simulink library "tp333079"  (Simulink 5.0)
values from neighbouring files (symbols this model uses):
  b = 1    [main_flock3.m]    (also in main_flock4.m; params_flocking_ros.m)
undefined symbols (not defined in the file or in its folder): AC, AlphaBnd, BetaBnd, CDda, CDde, CDdf, CDdr, CDM, CDmin, CGempty, CGgross, CL0, CLa, CLalphadot, Clbeta, Clda, CLde, CLdf, Cldr, CLM, CLmind, Clp, CLq, Clr, Cm0, Cma, Cmalphadot, Cmde, Cmdf, CmM, Cmq, Cnbeta, Cnda, Cndr, Cnp, Cnr, CP, CT, CYbeta, CYda, CYdr, CYp, CYr, Displacement, dmy, Engine, EulerIni, FuelFlow, FuelIni, J, Jempty, Jeng, Jgross, Jprop, MAC, MAP, MAPLim, MassIni, MaxPower, mempty ... (+26)
libraries: aerosimlib x325, simulink3 x42
(part 8 of 11)

== system tp333079/Unit Conversion/Pressure/inHg2Pa ==
  inHg : Inport  Port=1  PortDimensions=-1  SampleTime=-1  DataType=auto
      settings: SignalType=auto
  Gain : Gain  Gain=1/0.00029529  Multiplication=Element-wise(K.*u)  SaturateOnIntegerOverflow=on
  Pa : Outport  Port=1
  wires:
  inHg/1 -> Gain/1
  Gain/1 -> Pa/1

== system tp333079/Unit Conversion/Temperature/F2K ==
  F : Inport  Port=1  PortDimensions=-1  SampleTime=-1  DataType=auto
      settings: SignalType=auto
  Constant : Constant  Value=459.67
  Gain : Gain  Gain=1/1.8  Multiplication=Element-wise(K.*u)  SaturateOnIntegerOverflow=on
  Sum : Sum  Inputs=|++  SaturateOnIntegerOverflow=on
  K : Outport  Port=1
  wires:
  Constant/1 -> Sum/2
  F/1 -> Sum/1
  Sum/1 -> Gain/1
  Gain/1 -> K/1

== system tp333079/Unit Conversion/Temperature/K2F ==
  K : Inport  Port=1  PortDimensions=-1  SampleTime=-1  DataType=auto
      settings: SignalType=auto
  Constant : Constant  Value=459.67
  Gain : Gain  Gain=1.8  Multiplication=Element-wise(K.*u)  SaturateOnIntegerOverflow=on
  Sum : Sum  Inputs=|+-  SaturateOnIntegerOverflow=on
  F : Outport  Port=1
  wires:
  K/1 -> Gain/1
  Gain/1 -> Sum/1
  Constant/1 -> Sum/2
  Sum/1 -> F/1

== system tp333079/Unit Conversion/Velocity/km/h 2 m/s ==
  In : Inport  Port=1  PortDimensions=-1  SampleTime=-1  DataType=auto
      settings: SignalType=auto
  Gain : Gain  Gain=1/3.6  Multiplication=Element-wise(K.*u)  SaturateOnIntegerOverflow=on
  Out : Outport  Port=1
  wires:
  Gain/1 -> Out/1
  In/1 -> Gain/1

== system tp333079/Unit Conversion/Velocity/kts 2 m/s ==
  In : Inport  Port=1  PortDimensions=-1  SampleTime=-1  DataType=auto
      settings: SignalType=auto
  Gain : Gain  Gain=0.5147902667  Multiplication=Element-wise(K.*u)  SaturateOnIntegerOverflow=on
  Out : Outport  Port=1
  wires:
  Gain/1 -> Out/1
  In/1 -> Gain/1

== system tp333079/Unit Conversion/Velocity/m/s 2 km/h ==
  In : Inport  Port=1  PortDimensions=-1  SampleTime=-1  DataType=auto
      settings: SignalType=auto
  Gain : Gain  Gain=3.6  Multiplication=Element-wise(K.*u)  SaturateOnIntegerOverflow=on
  Out : Outport  Port=1
  wires:
  In/1 -> Gain/1
  Gain/1 -> Out/1

== system tp333079/Unit Conversion/Velocity/m/s 2 kts ==
  In : Inport  Port=1  PortDimensions=-1  SampleTime=-1  DataType=auto
      settings: SignalType=auto
  Gain : Gain  Gain=1.9425386701  Multiplication=Element-wise(K.*u)  SaturateOnIntegerOverflow=on
  Out : Outport  Port=1
  wires:
  In/1 -> Gain/1
  Gain/1 -> Out/1

== system tp333079/Unit Conversion/Velocity/m/s 2 mph ==
  In : Inport  Port=1  PortDimensions=-1  SampleTime=-1  DataType=auto
      settings: SignalType=auto
  Gain : Gain  Gain=2.2369362921  Multiplication=Element-wise(K.*u)  SaturateOnIntegerOverflow=on
  Out : Outport  Port=1
  wires:
  Gain/1 -> Out/1
  In/1 -> Gain/1

== system tp333079/Unit Conversion/Velocity/mph 2 m/s ==
  In : Inport  Port=1  PortDimensions=-1  SampleTime=-1  DataType=auto
      settings: SignalType=auto
  Gain : Gain  Gain=0.44704  Multiplication=Element-wise(K.*u)  SaturateOnIntegerOverflow=on
  Out : Outport  Port=1
  wires:
  In/1 -> Gain/1
  Gain/1 -> Out/1

== system tp333079/Unit Conversion/Volume/gal 2 l ==
  In : Inport  Port=1  PortDimensions=-1  SampleTime=-1  DataType=auto
      settings: SignalType=auto
  Gain : Gain  Gain=3.785412  Multiplication=Element-wise(K.*u)  SaturateOnIntegerOverflow=on
  Out : Outport  Port=1
  wires:
  Gain/1 -> Out/1
  In/1 -> Gain/1

== system tp333079/Unit Conversion/Volume/l 2 gal ==
  In : Inport  Port=1  PortDimensions=-1  SampleTime=-1  DataType=auto
      settings: SignalType=auto
  Gain : Gain  Gain=1/3.785412  Multiplication=Element-wise(K.*u)  SaturateOnIntegerOverflow=on
  Out : Outport  Port=1
  wires:
  In/1 -> Gain/1
  Gain/1 -> Out/1

== system tp333079/Atmosphere/Turbulence/Turbulence Characteristics/Vector norm ==
  Vec : Inport  Port=1  PortDimensions=-1  SampleTime=-1  DataType=auto
      settings: SignalType=auto
  Dot Product : simulink3/Math/Dot Product
  Math Function : Math  Operator=sqrt  OutputSignalType=auto
  Mag : Outport  Port=1
  wires:
  Vec/1 -> Dot Product/1, Dot Product/2
  Dot Product/1 -> Math Function/1
  Math Function/1 -> Mag/1

== system tp333079/Atmosphere/Wind Shear/Zero Offset1/Non-zero Sign ==
  In : Inport  Port=1  PortDimensions=-1  SampleTime=-1  DataType=auto
      settings: SignalType=auto
  One : Constant  Value=1
  Relational Operator : RelationalOperator  Operator===
  Sign : Signum
  Switch : Switch  Threshold=1
  Zero : Constant  Value=0
  Out : Outport  Port=1
  wires:
  Zero/1 -> Relational Operator/2
  In/1 -> Relational Operator/1, Sign/1
  Relational Operator/1 -> Switch/2
  One/1 -> Switch/1
  Sign/1 -> Switch/3
  Switch/1 -> Out/1

== system tp333079/Atmosphere/Wind Shear/Zero Offset2/Non-zero Sign ==
  In : Inport  Port=1  PortDimensions=-1  SampleTime=-1  DataType=auto
      settings: SignalType=auto
  One : Constant  Value=1
  Relational Operator : RelationalOperator  Operator===
  Sign : Signum
  Switch : Switch  Threshold=1
  Zero : Constant  Value=0
  Out : Outport  Port=1
  wires:
  Switch/1 -> Out/1
  Sign/1 -> Switch/3
  One/1 -> Switch/1
  Relational Operator/1 -> Switch/2
  In/1 -> Sign/1, Relational Operator/1
  Zero/1 -> Relational Operator/2

== system tp333079/Equations of Motion/Body-Frame EOM/Kinematics (Quaternions)/Normalization ==
  VecIn : Inport  Port=1  PortDimensions=-1  SampleTime=-1  DataType=auto
      settings: SignalType=auto
  Vector norm : Subsystem  SimViewingDevice=off
      settings: Permissions=ReadWrite  RTWFcnNameOpts=Auto  RTWFileNameOpts=Auto
      mask Type: Vector norm-2
      mask Description: Compute the 2-norm (magnitude) of a vector, |v| = sqrt(v'v)
  e/|e| : Product  Inputs=*/  Multiplication=Element-wise(.*)  SaturateOnIntegerOverflow=on
  VecOut : Outport  Port=1
  wires:
  Vector norm/1(Mag) -> e/|e|/2
  e/|e|/1 -> VecOut/1
  VecIn/1 -> Vector norm/1(Vec), e/|e|/1

== system tp333079/Equations of Motion/Body-Frame EOM/Navigation/Latitude Bound ==
  In : Inport  Port=1  PortDimensions=-1  SampleTime=-1  DataType=auto
      settings: SignalType=auto
  2pi : Constant  Value=2*pi
  ChSign : Gain  Gain=-1  Multiplication=Element-wise(K.*u)  SaturateOnIntegerOverflow=on
  Math Function : Math  Operator=mod  OutputSignalType=auto
  Math Function1 : Math  Operator=mod  OutputSignalType=auto
  Sum1 : Sum  Inputs=|+-  SaturateOnIntegerOverflow=on
  Sum2 : Sum  Inputs=|++  SaturateOnIntegerOverflow=on
  Switch : Switch  Threshold=pi
  pi : Constant  Value=pi
  pi/2 : Constant  Value=pi/2
  Out : Outport  Port=1
  wires:
  2pi/1 -> Math Function1/2
  ChSign/1 -> Switch/1
  Sum2/1 -> Math Function1/1, Math Function/1
  In/1 -> Sum2/1
  Switch/1 -> Out/1
  Math Function1/1 -> Switch/2
  Sum1/1 -> Switch/3, ChSign/1
  pi/2/1 -> Sum2/2, Sum1/2
  Math Function/1 -> Sum1/1
  pi/1 -> Math Function/2

== system tp333079/Equations of Motion/Body-Frame EOM/Navigation/Longitude Bound ==
  In : Inport  Port=1  PortDimensions=-1  SampleTime=-1  DataType=auto
      settings: SignalType=auto
  2pi : Constant  Value=2*pi
  Math Function : Math  Operator=mod  OutputSignalType=auto
  Sum1 : Sum  Inputs=|+-  SaturateOnIntegerOverflow=on
  Sum2 : Sum  Inputs=|++  SaturateOnIntegerOverflow=on
  pi : Constant  Value=pi
  Out : Outport  Port=1
  wires:
  Math Function/1 -> Sum1/1
  2pi/1 -> Math Function/2
  In/1 -> Sum2/1
  Sum2/1 -> Math Function/1
  pi/1 -> Sum2/2, Sum1/2
  Sum1/1 -> Out/1

== system tp333079/Equations of Motion/Geodetic-Frame EOM/Position/Latitude Bound ==
  In : Inport  Port=1  PortDimensions=-1  SampleTime=-1  DataType=auto
      settings: SignalType=auto
  2pi : Constant  Value=2*pi
  ChSign : Gain  Gain=-1  Multiplication=Element-wise(K.*u)  SaturateOnIntegerOverflow=on
  Math Function : Math  Operator=mod  OutputSignalType=auto
  Math Function1 : Math  Operator=mod  OutputSignalType=auto
  Sum1 : Sum  Inputs=|+-  SaturateOnIntegerOverflow=on
  Sum2 : Sum  Inputs=|++  SaturateOnIntegerOverflow=on
  Switch : Switch  Threshold=pi
  pi : Constant  Value=pi
  pi/2 : Constant  Value=pi/2
  Out : Outport  Port=1
  wires:
  pi/1 -> Math Function/2
  Math Function/1 -> Sum1/1
  pi/2/1 -> Sum1/2, Sum2/2
  Sum1/1 -> ChSign/1, Switch/3
  Math Function1/1 -> Switch/2
  Switch/1 -> Out/1
  In/1 -> Sum2/1
  Sum2/1 -> Math Function/1, Math Function1/1
  ChSign/1 -> Switch/1
  2pi/1 -> Math Function1/2

== system tp333079/Equations of Motion/Geodetic-Frame EOM/Position/Longitude Bound ==
  In : Inport  Port=1  PortDimensions=-1  SampleTime=-1  DataType=auto
      settings: SignalType=auto
  2pi : Constant  Value=2*pi
  Math Function : Math  Operator=mod  OutputSignalType=auto
  Sum1 : Sum  Inputs=|+-  SaturateOnIntegerOverflow=on
  Sum2 : Sum  Inputs=|++  SaturateOnIntegerOverflow=on
  pi : Constant  Value=pi
  Out : Outport  Port=1
  wires:
  Sum1/1 -> Out/1
  pi/1 -> Sum1/2, Sum2/2
  Sum2/1 -> Math Function/1
  In/1 -> Sum2/1
  2pi/1 -> Math Function/2
  Math Function/1 -> Sum1/1

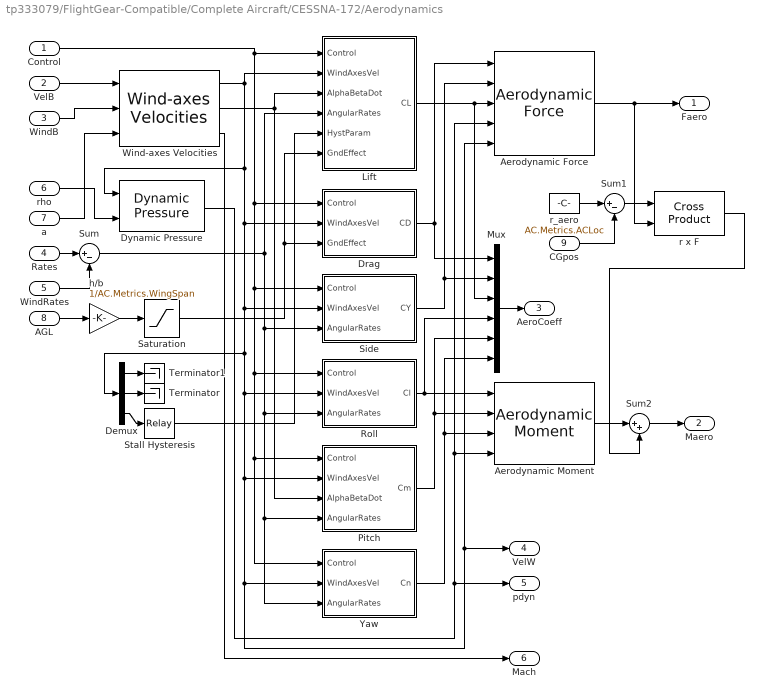
== system tp333079/FlightGear-Compatible/Complete Aircraft/CESSNA-172/Aerodynamics ==
  Control : Inport  Port=1  PortDimensions=[4 1]  SampleTime=-1  DataType=auto
      settings: SignalType=auto
  VelB : Inport  Port=2  PortDimensions=[3 1]  SampleTime=-1  DataType=auto
      settings: SignalType=auto
  WindB : Inport  Port=3  PortDimensions=[3 1]  SampleTime=-1  DataType=auto
      settings: SignalType=auto
  Rates : Inport  Port=4  PortDimensions=[3 1]  SampleTime=-1  DataType=auto
      settings: SignalType=auto
  WindRates : Inport  Port=5  PortDimensions=[3 1]  SampleTime=-1  DataType=auto
      settings: SignalType=auto
  rho : Inport  Port=6  PortDimensions=1  SampleTime=-1  DataType=auto
      settings: SignalType=auto
  a : Inport  Port=7  PortDimensions=1  SampleTime=-1  DataType=auto
      settings: SignalType=auto
  AGL : Inport  Port=8  PortDimensions=1  SampleTime=-1  DataType=auto
      settings: SignalType=auto
  CGpos : Inport  Port=9  PortDimensions=[3 1]  SampleTime=-1  DataType=auto
      settings: SignalType=auto
  Aerodynamic Force : aerosimlib/Aerodynamics/Aerodynamic Force  S=AC.Metrics.WingArea
  Aerodynamic Moment : aerosimlib/Aerodynamics/Aerodynamic Moment  c=AC.Metrics.WingChord  b=AC.Metrics.WingSpan  S=AC.Metrics.WingArea
  Demux : Demux  Outputs=3  BusSelectionMode=off
  Drag : Subsystem  SimViewingDevice=off
      settings: Permissions=ReadWrite  RTWFcnNameOpts=Auto  RTWFileNameOpts=Auto
  Dynamic Pressure : aerosimlib/Aerodynamics/Dynamic Pressure
  Lift : Subsystem  SimViewingDevice=off
      settings: Permissions=ReadWrite  RTWFcnNameOpts=Auto  RTWFileNameOpts=Auto
  Mux : Mux  Inputs=6
  Pitch : Subsystem  SimViewingDevice=off
      settings: Permissions=ReadWrite  RTWFcnNameOpts=Auto  RTWFileNameOpts=Auto
  Roll : Subsystem  SimViewingDevice=off
      settings: Permissions=ReadWrite  RTWFcnNameOpts=Auto  RTWFileNameOpts=Auto
  Saturation : Saturate  UpperLimit=1  LowerLimit=0  LinearizeAsGain=on
  Side : Subsystem  SimViewingDevice=off
      settings: Permissions=ReadWrite  RTWFcnNameOpts=Auto  RTWFileNameOpts=Auto
  Stall Hysteresis : Relay  OnSwitchValue=AC.Aerodynamics.HystLim(2)  OffSwitchValue=AC.Aerodynamics.HystLim(1)  OnOutputValue=1  OffOutputValue=0
  Sum : Sum  Inputs=|+-  SaturateOnIntegerOverflow=on
  Sum1 : Sum  Inputs=|+-  SaturateOnIntegerOverflow=on
  Sum2 : Sum  Inputs=|++  SaturateOnIntegerOverflow=on
  Terminator : Terminator
  Terminator1 : Terminator
  Wind-axes Velocities : aerosimlib/Aerodynamics/Wind-axes Velocities  Vabnd=[0 1000]  betabnd=[-1 1]  alphabnd=AC.Aerodynamics.AlphaLim
  Yaw : Subsystem  SimViewingDevice=off
      settings: Permissions=ReadWrite  RTWFcnNameOpts=Auto  RTWFileNameOpts=Auto
  h/b : Gain  Gain=1/AC.Metrics.WingSpan  Multiplication=Element-wise(K.*u)  SaturateOnIntegerOverflow=on
  r x F : aerosimlib/Math/Cross Product
  r_aero : Constant  Value=AC.Metrics.ACLoc
  Faero : Outport  Port=1
  Maero : Outport  Port=2
  AeroCoeff : Outport  Port=3
  VelW : Outport  Port=4
  pdyn : Outport  Port=5
  Mach : Outport  Port=6
  wires:
  Sum/1 -> Yaw/3(AngularRates), Pitch/4(AngularRates), Roll/3(AngularRates), Side/3(AngularRates), Lift/4(AngularRates)
  WindRates/1 -> Sum/2
  Rates/1 -> Sum/1
  Stall Hysteresis/1 -> Lift/5(HystParam)
  Demux/2 -> Terminator/1
  Demux/1 -> Terminator1/1
  Demux/3 -> Stall Hysteresis/1
  Saturation/1 -> Drag/3(GndEffect), Lift/6(GndEffect)
  AGL/1 -> h/b/1
  h/b/1 -> Saturation/1
  Wind-axes Velocities/3 -> Mach/1
  Yaw/1(Cn) -> Mux/6, Aerodynamic Moment/3
  Pitch/1(Cm) -> Mux/5, Aerodynamic Moment/2
  Roll/1(Cl) -> Mux/4, Aerodynamic Moment/1
  Dynamic Pressure/1 -> pdyn/1, Aerodynamic Moment/4, Aerodynamic Force/4
  Side/1(CY) -> Mux/2, Aerodynamic Force/2
  Drag/1(CD) -> Mux/1, Aerodynamic Force/1
  Lift/1(CL) -> Mux/3, Aerodynamic Force/3
  Wind-axes Velocities/2 -> Lift/3(AlphaBetaDot), Pitch/3(AlphaBetaDot)
  Control/1 -> Pitch/1(Control), Yaw/1(Control), Roll/1(Control), Side/1(Control), Drag/1(Control), Lift/1(Control)
  Wind-axes Velocities/1 -> Lift/2(WindAxesVel), Demux/1, VelW/1, Aerodynamic Force/5, Yaw/2(WindAxesVel), Pitch/2(WindAxesVel), Roll/2(WindAxesVel), Side/2(WindAxesVel), Drag/2(WindAxesVel), Dynamic Pressure/1
  rho/1 -> Dynamic Pressure/2
  a/1 -> Wind-axes Velocities/3
  WindB/1 -> Wind-axes Velocities/2
  VelB/1 -> Wind-axes Velocities/1
  Mux/1 -> AeroCoeff/1
  CGpos/1 -> Sum1/2
  r_aero/1 -> Sum1/1
  Sum1/1 -> r x F/1
  Aerodynamic Force/1 -> Faero/1, r x F/2
  Aerodynamic Moment/1 -> Sum2/1
  Sum2/1 -> Maero/1
  r x F/1 -> Sum2/2

== system tp333079/FlightGear-Compatible/Complete Aircraft/CESSNA-172/Aircraft Inertia ==
  FuelFlow : Inport  Port=1  PortDimensions=-1  SampleTime=-1  DataType=auto
      settings: SignalType=auto
  RST : Inport  Port=2  PortDimensions=-1  SampleTime=-1  DataType=auto
      settings: SignalType=auto
  1/2 : Gain  Gain=1/2  Multiplication=Element-wise(K.*u)  SaturateOnIntegerOverflow=on
  Empty Aircraft : aerosimlib/FlightGear-Compatible/Inertia/Empty Aircraft  Metrics=AC.Metrics
  Left Wing Tank : aerosimlib/FlightGear-Compatible/Propulsion/Tank/Fuel Tank  MassIni=FuelIni(1)  Tank=AC.Propulsion.Tank{1}
  Pilot Point Mass : aerosimlib/FlightGear-Compatible/Inertia/Point Mass  PointMass=AC.Metrics.PointMass{1}
  Product{,1..3} (4 alike) : Product  Inputs=2  Multiplication=Element-wise(.*)  SaturateOnIntegerOverflow=on
  Product4 : Product  Inputs=*/  Multiplication=Element-wise(.*)  SaturateOnIntegerOverflow=on
  Right Wing Tank : aerosimlib/FlightGear-Compatible/Propulsion/Tank/Fuel Tank  MassIni=FuelIni(2)  Tank=AC.Propulsion.Tank{2}
  Sum1 : Sum  Inputs=++++  SaturateOnIntegerOverflow=on
  Sum2 : Sum  Inputs=++++  SaturateOnIntegerOverflow=on
  Sum3 : Sum  Inputs=++++  SaturateOnIntegerOverflow=on
  Mass : Outport  Port=1
  CG : Outport  Port=2
  Inertia : Outport  Port=3
  wires:
  Sum3/1 -> Inertia/1
  Right Wing Tank/3 -> Sum3/4
  Left Wing Tank/3 -> Sum3/3
  Pilot Point Mass/3 -> Sum3/2
  Empty Aircraft/3 -> Sum3/1
  Product4/1 -> CG/1
  Sum1/1 -> Product4/1
  Product2/1 -> Sum1/4
  Product1/1 -> Sum1/3
  Product/1 -> Sum1/2
  Product3/1 -> Sum1/1
  Empty Aircraft/2 -> Product3/2
  Right Wing Tank/2 -> Product2/2
  Left Wing Tank/2 -> Product1/2
  Pilot Point Mass/2 -> Product/2
  Right Wing Tank/1 -> Product2/1, Sum2/4
  Left Wing Tank/1 -> Product1/1, Sum2/3
  Pilot Point Mass/1 -> Product/1, Sum2/2
  Empty Aircraft/1 -> Product3/1, Sum2/1
  Sum2/1 -> Product4/2, Mass/1
  RST/1 -> Right Wing Tank/2, Left Wing Tank/2
  FuelFlow/1 -> 1/2/1
  1/2/1 -> Right Wing Tank/1, Left Wing Tank/1

== system tp333079/FlightGear-Compatible/Complete Aircraft/CESSNA-172/Atmosphere ==
  note: Inputs
  note: Outputs
  MSL : Inport  Port=1  PortDimensions=1  SampleTime=-1  DataType=double
      settings: SignalType=auto
  AGL : Inport  Port=2  PortDimensions=1  SampleTime=-1  DataType=double
      settings: SignalType=auto
  Winds : Inport  Port=3  PortDimensions=[3 1]  SampleTime=-1  DataType=double
      settings: SignalType=auto
  VelB : Inport  Port=4  PortDimensions=[3 1]  SampleTime=-1  DataType=double
      settings: SignalType=auto
  VelW : Inport  Port=5  PortDimensions=[3 1]  SampleTime=-1  DataType=auto
      settings: SignalType=auto
  DCM : Inport  Port=6  PortDimensions=[3 3]  SampleTime=-1  DataType=double
      settings: SignalType=auto
  Background Wind : aerosimlib/Atmosphere/Background Wind
  Standard Atmosphere : aerosimlib/Atmosphere/Standard Atmosphere
  Sum : Sum  Inputs=|++  SaturateOnIntegerOverflow=on
  Turbulence : aerosimlib/Atmosphere/Turbulence  tsamp=tsamp
  Wind Shear : aerosimlib/Atmosphere/Wind Shear
  pstatic : Outport  Port=1
  OAT : Outport  Port=2
  rho : Outport  Port=3
  a : Outport  Port=4
  WindVel : Outport  Port=5
  WindRates : Outport  Port=6
  wires:
  MSL/1 -> Standard Atmosphere/1
  Winds/1 -> Background Wind/1
  DCM/1 -> Background Wind/2
  Background Wind/1 -> Turbulence/3, Sum/2
  AGL/1 -> Turbulence/2
  VelW/1 -> Turbulence/1
  Background Wind/2 -> Wind Shear/1
  Turbulence/1 -> Sum/1
  Turbulence/2 -> Wind Shear/2
  VelB/1 -> Wind Shear/3
  Wind Shear/1 -> WindRates/1
  Standard Atmosphere/1 -> pstatic/1
  Standard Atmosphere/2 -> OAT/1
  Standard Atmosphere/3 -> rho/1
  Standard Atmosphere/4 -> a/1
  Sum/1 -> WindVel/1

== system tp333079/FlightGear-Compatible/Complete Aircraft/CESSNA-172/Earth ==
  note: Inputs
  note: Outputs
  Position : Inport  Port=1  PortDimensions=[3 1]  SampleTime=-1  DataType=double
      settings: SignalType=auto
  EGM-96 : aerosimlib/Earth/EGM-96
  Ground Alt : Constant  Value=GndAlt
  Ground Detection : aerosimlib/Earth/Ground Detection
  Mux3 : Mux  Inputs=2
  WGS-84 : aerosimlib/Earth/WGS-84
  MSL : Outport  Port=1
  AGL : Outport  Port=2
  AConGnd : Outport  Port=3
  Rearth : Outport  Port=4
  Requiv : Outport  Port=5
  Gravity : Outport  Port=6
  wires:
  Position/1 -> EGM-96/1, WGS-84/1
  Ground Alt/1 -> Ground Detection/2
  EGM-96/1 -> Ground Detection/1, MSL/1
  WGS-84/1 -> Mux3/1
  WGS-84/2 -> Mux3/2
  Ground Detection/2 -> AGL/1
  Ground Detection/1 -> AConGnd/1
  Mux3/1 -> Rearth/1
  WGS-84/3 -> Requiv/1
  WGS-84/4 -> Gravity/1

== system tp333079/FlightGear-Compatible/Complete Aircraft/CESSNA-172/Equations of Motion ==
  note: Inputs
  note: Outputs
  Accel : Inport  Port=1  PortDimensions=[3 1]  SampleTime=-1  DataType=auto
      settings: SignalType=auto
  Moment : Inport  Port=2  PortDimensions=[3 1]  SampleTime=-1  DataType=auto
      settings: SignalType=auto
  Inertia : Inport  Port=3  PortDimensions=[4 1]  SampleTime=-1  DataType=auto
      settings: SignalType=auto
  Rearth : Inport  Port=4  PortDimensions=[2 1]  SampleTime=-1  DataType=auto
      settings: SignalType=auto
  Gravity : Inport  Port=5  PortDimensions=1  SampleTime=-1  DataType=auto
      settings: SignalType=auto
  AConGnd : Inport  Port=6  PortDimensions=1  SampleTime=-1  DataType=auto
      settings: SignalType=auto
  RST : Inport  Port=7  PortDimensions=1  SampleTime=-1  DataType=auto
      settings: SignalType=auto
  Angular Rate : aerosimlib/Equations of Motion/Geodetic-Frame EOM/Angular Rate  RatesIni=RatesIni
  Attitude (Quaternions) : aerosimlib/Equations of Motion/Body-Frame EOM/Kinematics (Quaternions)  QuaternionsIni=QuaternionsIni
  Body-Inertial DCM From Quaternions : aerosimlib/Transformations/Body-Inertial DCM From Quaternions
  Demux : Demux  Outputs=2  BusSelectionMode=off
  Euler Angles From Quaternions : aerosimlib/Transformations/Euler Angles From Quaternions
  Position : aerosimlib/Equations of Motion/Geodetic-Frame EOM/Position  PositionIni=PositionIni
  Product : Product  Inputs=2  Multiplication=Matrix(*)  SaturateOnIntegerOverflow=on
  Velocity : aerosimlib/Equations of Motion/Geodetic-Frame EOM/Velocity  VelocitiesIni=VelocitiesIni
  VelB : Outport  Port=1
  VelNED : Outport  Port=2
  Rates : Outport  Port=3
  Quaternions : Outport  Port=4
  Pos : Outport  Port=5
  DCM : Outport  Port=6
  Euler : Outport  Port=7
  Ang Acc : Outport  Port=8
  wires:
  Attitude (Quaternions)/1 -> Quaternions/1, Euler Angles From Quaternions/1, Body-Inertial DCM From Quaternions/1
  Position/1 -> Velocity/1, Angular Rate/3, Pos/1
  Position/2 -> Velocity/2, Angular Rate/4
  Velocity/1 -> Product/2, Position/1, VelNED/1
  Demux/1 -> Position/2
  Demux/2 -> Position/3
  Rearth/1 -> Demux/1
  Gravity/1 -> Velocity/5
  RST/1 -> Velocity/6, Position/5, Angular Rate/6, Attitude (Quaternions)/2
  Angular Rate/1 -> Rates/1, Attitude (Quaternions)/1
  Moment/1 -> Angular Rate/2
  Inertia/1 -> Angular Rate/1
  Body-Inertial DCM From Quaternions/1 -> Angular Rate/5, Velocity/4, Product/1, DCM/1
  AConGnd/1 -> Position/4
  Accel/1 -> Velocity/3
  Product/1 -> VelB/1
  Angular Rate/2 -> Ang Acc/1
  Euler Angles From Quaternions/1 -> Euler/1

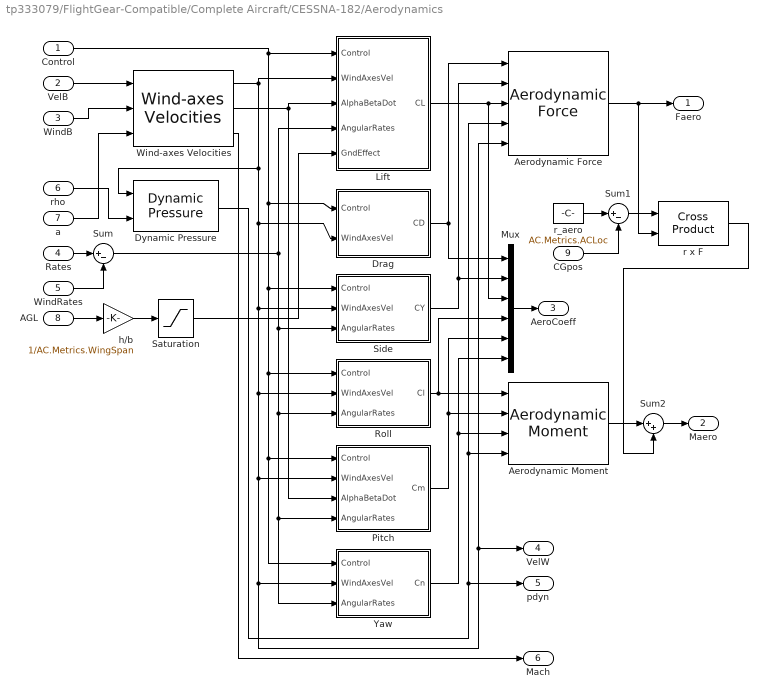
== system tp333079/FlightGear-Compatible/Complete Aircraft/CESSNA-182/Aerodynamics ==
  Control : Inport  Port=1  PortDimensions=[4 1]  SampleTime=-1  DataType=auto
      settings: SignalType=auto
  VelB : Inport  Port=2  PortDimensions=[3 1]  SampleTime=-1  DataType=auto
      settings: SignalType=auto
  WindB : Inport  Port=3  PortDimensions=[3 1]  SampleTime=-1  DataType=auto
      settings: SignalType=auto
  Rates : Inport  Port=4  PortDimensions=[3 1]  SampleTime=-1  DataType=auto
      settings: SignalType=auto
  WindRates : Inport  Port=5  PortDimensions=[3 1]  SampleTime=-1  DataType=auto
      settings: SignalType=auto
  rho : Inport  Port=6  PortDimensions=1  SampleTime=-1  DataType=auto
      settings: SignalType=auto
  a : Inport  Port=7  PortDimensions=1  SampleTime=-1  DataType=auto
      settings: SignalType=auto
  AGL : Inport  Port=8  PortDimensions=1  SampleTime=-1  DataType=auto
      settings: SignalType=auto
  CGpos : Inport  Port=9  PortDimensions=[3 1]  SampleTime=-1  DataType=auto
      settings: SignalType=auto
  Aerodynamic Force : aerosimlib/Aerodynamics/Aerodynamic Force  S=AC.Metrics.WingArea
  Aerodynamic Moment : aerosimlib/Aerodynamics/Aerodynamic Moment  c=AC.Metrics.WingChord  b=AC.Metrics.WingSpan  S=AC.Metrics.WingArea
  Drag : Subsystem  SimViewingDevice=off
      settings: Permissions=ReadWrite  RTWFcnNameOpts=Auto  RTWFileNameOpts=Auto
  Dynamic Pressure : aerosimlib/Aerodynamics/Dynamic Pressure
  Lift : Subsystem  SimViewingDevice=off
      settings: Permissions=ReadWrite  RTWFcnNameOpts=Auto  RTWFileNameOpts=Auto
  Mux : Mux  Inputs=6
  Pitch : Subsystem  SimViewingDevice=off
      settings: Permissions=ReadWrite  RTWFcnNameOpts=Auto  RTWFileNameOpts=Auto
  Roll : Subsystem  SimViewingDevice=off
      settings: Permissions=ReadWrite  RTWFcnNameOpts=Auto  RTWFileNameOpts=Auto
  Saturation : Saturate  UpperLimit=1  LowerLimit=0  LinearizeAsGain=on
  Side : Subsystem  SimViewingDevice=off
      settings: Permissions=ReadWrite  RTWFcnNameOpts=Auto  RTWFileNameOpts=Auto
  Sum : Sum  Inputs=|+-  SaturateOnIntegerOverflow=on
  Sum1 : Sum  Inputs=|+-  SaturateOnIntegerOverflow=on
  Sum2 : Sum  Inputs=|++  SaturateOnIntegerOverflow=on
  Wind-axes Velocities : aerosimlib/Aerodynamics/Wind-axes Velocities  Vabnd=[0 1000]  betabnd=[-1 1]  alphabnd=AC.Aerodynamics.AlphaLim
  Yaw : Subsystem  SimViewingDevice=off
      settings: Permissions=ReadWrite  RTWFcnNameOpts=Auto  RTWFileNameOpts=Auto
  h/b : Gain  Gain=1/AC.Metrics.WingSpan  Multiplication=Element-wise(K.*u)  SaturateOnIntegerOverflow=on
  r x F : aerosimlib/Math/Cross Product
  r_aero : Constant  Value=AC.Metrics.ACLoc
  Faero : Outport  Port=1
  Maero : Outport  Port=2
  AeroCoeff : Outport  Port=3
  VelW : Outport  Port=4
  pdyn : Outport  Port=5
  Mach : Outport  Port=6
  wires:
  Rates/1 -> Sum/1
  Sum/1 -> Yaw/3(AngularRates), Pitch/4(AngularRates), Roll/3(AngularRates), Side/3(AngularRates), Lift/4(AngularRates)
  WindRates/1 -> Sum/2
  Saturation/1 -> Lift/5(GndEffect)
  AGL/1 -> h/b/1
  h/b/1 -> Saturation/1
  Wind-axes Velocities/3 -> Mach/1
  Aerodynamic Force/1 -> Faero/1, r x F/2
  Yaw/1(Cn) -> Mux/6, Aerodynamic Moment/3
  Pitch/1(Cm) -> Mux/5, Aerodynamic Moment/2
  Roll/1(Cl) -> Mux/4, Aerodynamic Moment/1
  Dynamic Pressure/1 -> pdyn/1, Aerodynamic Moment/4, Aerodynamic Force/4
  Side/1(CY) -> Mux/2, Aerodynamic Force/2
  Drag/1(CD) -> Mux/1, Aerodynamic Force/1
  Lift/1(CL) -> Mux/3, Aerodynamic Force/3
  Wind-axes Velocities/2 -> Lift/3(AlphaBetaDot), Pitch/3(AlphaBetaDot)
  Control/1 -> Pitch/1(Control), Yaw/1(Control), Roll/1(Control), Side/1(Control), Drag/1(Control), Lift/1(Control)
  Wind-axes Velocities/1 -> Lift/2(WindAxesVel), VelW/1, Aerodynamic Force/5, Yaw/2(WindAxesVel), Pitch/2(WindAxesVel), Roll/2(WindAxesVel), Side/2(WindAxesVel), Drag/2(WindAxesVel), Dynamic Pressure/1
  rho/1 -> Dynamic Pressure/2
  a/1 -> Wind-axes Velocities/3
  WindB/1 -> Wind-axes Velocities/2
  VelB/1 -> Wind-axes Velocities/1
  Mux/1 -> AeroCoeff/1
  CGpos/1 -> Sum1/2
  r_aero/1 -> Sum1/1
  Sum1/1 -> r x F/1
  Aerodynamic Moment/1 -> Sum2/1
  Sum2/1 -> Maero/1
  r x F/1 -> Sum2/2

== system tp333079/FlightGear-Compatible/Complete Aircraft/CESSNA-182/Aircraft Inertia ==
  FuelFlow : Inport  Port=1  PortDimensions=-1  SampleTime=-1  DataType=auto
      settings: SignalType=auto
  RST : Inport  Port=2  PortDimensions=-1  SampleTime=-1  DataType=auto
      settings: SignalType=auto
  1/2 : Gain  Gain=1/2  Multiplication=Element-wise(K.*u)  SaturateOnIntegerOverflow=on
  Empty Aircraft : aerosimlib/FlightGear-Compatible/Inertia/Empty Aircraft  Metrics=AC.Metrics
  Left Wing Tank : aerosimlib/FlightGear-Compatible/Propulsion/Tank/Fuel Tank  MassIni=FuelIni(1)  Tank=AC.Propulsion.Tank{1}
  Pilot Point Mass : aerosimlib/FlightGear-Compatible/Inertia/Point Mass  PointMass=AC.Metrics.PointMass{1}
  Product{,1..3} (4 alike) : Product  Inputs=2  Multiplication=Element-wise(.*)  SaturateOnIntegerOverflow=on
  Product4 : Product  Inputs=*/  Multiplication=Element-wise(.*)  SaturateOnIntegerOverflow=on
  Right Wing Tank : aerosimlib/FlightGear-Compatible/Propulsion/Tank/Fuel Tank  MassIni=FuelIni(2)  Tank=AC.Propulsion.Tank{2}
  Sum1 : Sum  Inputs=++++  SaturateOnIntegerOverflow=on
  Sum2 : Sum  Inputs=++++  SaturateOnIntegerOverflow=on
  Sum3 : Sum  Inputs=++++  SaturateOnIntegerOverflow=on
  Mass : Outport  Port=1
  CG : Outport  Port=2
  Inertia : Outport  Port=3
  wires:
  Sum3/1 -> Inertia/1
  Right Wing Tank/3 -> Sum3/4
  Left Wing Tank/3 -> Sum3/3
  Pilot Point Mass/3 -> Sum3/2
  Empty Aircraft/3 -> Sum3/1
  Product4/1 -> CG/1
  Sum1/1 -> Product4/1
  Product2/1 -> Sum1/4
  Product1/1 -> Sum1/3
  Product/1 -> Sum1/2
  Product3/1 -> Sum1/1
  Empty Aircraft/2 -> Product3/2
  Right Wing Tank/2 -> Product2/2
  Left Wing Tank/2 -> Product1/2
  Pilot Point Mass/2 -> Product/2
  Right Wing Tank/1 -> Product2/1, Sum2/4
  Left Wing Tank/1 -> Product1/1, Sum2/3
  Pilot Point Mass/1 -> Product/1, Sum2/2
  Empty Aircraft/1 -> Product3/1, Sum2/1
  Sum2/1 -> Product4/2, Mass/1
  RST/1 -> Right Wing Tank/2, Left Wing Tank/2
  FuelFlow/1 -> 1/2/1
  1/2/1 -> Right Wing Tank/1, Left Wing Tank/1

== system tp333079/FlightGear-Compatible/Complete Aircraft/CESSNA-182/Earth ==
  note: Inputs
  note: Outputs
  Position : Inport  Port=1  PortDimensions=[3 1]  SampleTime=-1  DataType=double
      settings: SignalType=auto
  EGM-96 : aerosimlib/Earth/EGM-96
  Ground Alt : Constant  Value=GndAlt
  Ground Detection : aerosimlib/Earth/Ground Detection
  Mux3 : Mux  Inputs=2
  WGS-84 : aerosimlib/Earth/WGS-84
  MSL : Outport  Port=1
  AGL : Outport  Port=2
  AConGnd : Outport  Port=3
  Rearth : Outport  Port=4
  Requiv : Outport  Port=5
  Gravity : Outport  Port=6
  wires:
  Position/1 -> EGM-96/1, WGS-84/1
  Ground Alt/1 -> Ground Detection/2
  EGM-96/1 -> Ground Detection/1, MSL/1
  WGS-84/1 -> Mux3/1
  WGS-84/2 -> Mux3/2
  Ground Detection/2 -> AGL/1
  Ground Detection/1 -> AConGnd/1
  Mux3/1 -> Rearth/1
  WGS-84/3 -> Requiv/1
  WGS-84/4 -> Gravity/1

== system tp333079/FlightGear-Compatible/Complete Aircraft/CESSNA-182/Equations of Motion ==
  note: Inputs
  note: Outputs
  Accel : Inport  Port=1  PortDimensions=[3 1]  SampleTime=-1  DataType=auto
      settings: SignalType=auto
  Moment : Inport  Port=2  PortDimensions=[3 1]  SampleTime=-1  DataType=auto
      settings: SignalType=auto
  Inertia : Inport  Port=3  PortDimensions=[4 1]  SampleTime=-1  DataType=auto
      settings: SignalType=auto
  Rearth : Inport  Port=4  PortDimensions=[2 1]  SampleTime=-1  DataType=auto
      settings: SignalType=auto
  Gravity : Inport  Port=5  PortDimensions=1  SampleTime=-1  DataType=auto
      settings: SignalType=auto
  AConGnd : Inport  Port=6  PortDimensions=1  SampleTime=-1  DataType=auto
      settings: SignalType=auto
  RST : Inport  Port=7  PortDimensions=1  SampleTime=-1  DataType=auto
      settings: SignalType=auto
  Angular Rate : aerosimlib/Equations of Motion/Geodetic-Frame EOM/Angular Rate  RatesIni=RatesIni
  Attitude (Quaternions) : aerosimlib/Equations of Motion/Body-Frame EOM/Kinematics (Quaternions)  QuaternionsIni=QuaternionsIni
  Body-Inertial DCM From Quaternions : aerosimlib/Transformations/Body-Inertial DCM From Quaternions
  Demux : Demux  Outputs=2  BusSelectionMode=off
  Euler Angles From Quaternions : aerosimlib/Transformations/Euler Angles From Quaternions
  Position : aerosimlib/Equations of Motion/Geodetic-Frame EOM/Position  PositionIni=PositionIni
  Product : Product  Inputs=2  Multiplication=Matrix(*)  SaturateOnIntegerOverflow=on
  Velocity : aerosimlib/Equations of Motion/Geodetic-Frame EOM/Velocity  VelocitiesIni=VelocitiesIni
  VelB : Outport  Port=1
  VelNED : Outport  Port=2
  Rates : Outport  Port=3
  Quaternions : Outport  Port=4
  Pos : Outport  Port=5
  DCM : Outport  Port=6
  Euler : Outport  Port=7
  Ang Acc : Outport  Port=8
  wires:
  Attitude (Quaternions)/1 -> Quaternions/1, Euler Angles From Quaternions/1, Body-Inertial DCM From Quaternions/1
  Position/1 -> Velocity/1, Angular Rate/3, Pos/1
  Position/2 -> Velocity/2, Angular Rate/4
  Velocity/1 -> Product/2, Position/1, VelNED/1
  Demux/1 -> Position/2
  Demux/2 -> Position/3
  Rearth/1 -> Demux/1
  Gravity/1 -> Velocity/5
  RST/1 -> Velocity/6, Position/5, Angular Rate/6, Attitude (Quaternions)/2
  Angular Rate/1 -> Rates/1, Attitude (Quaternions)/1
  Moment/1 -> Angular Rate/2
  Inertia/1 -> Angular Rate/1
  Body-Inertial DCM From Quaternions/1 -> Angular Rate/5, Velocity/4, Product/1, DCM/1
  AConGnd/1 -> Position/4
  Accel/1 -> Velocity/3
  Product/1 -> VelB/1
  Angular Rate/2 -> Ang Acc/1
  Euler Angles From Quaternions/1 -> Euler/1

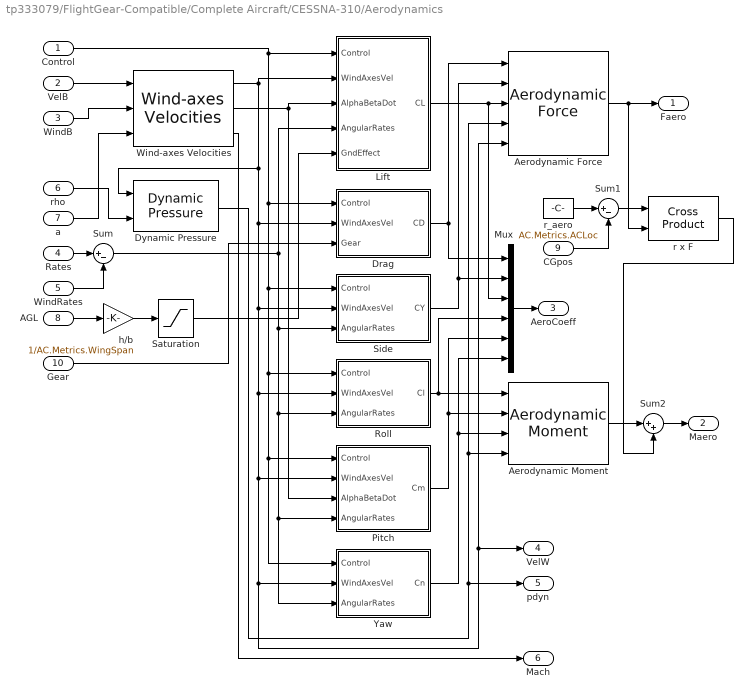
== system tp333079/FlightGear-Compatible/Complete Aircraft/CESSNA-310/Aerodynamics ==
  Control : Inport  Port=1  PortDimensions=[4 1]  SampleTime=-1  DataType=auto
      settings: SignalType=auto
  VelB : Inport  Port=2  PortDimensions=[3 1]  SampleTime=-1  DataType=auto
      settings: SignalType=auto
  WindB : Inport  Port=3  PortDimensions=[3 1]  SampleTime=-1  DataType=auto
      settings: SignalType=auto
  Rates : Inport  Port=4  PortDimensions=[3 1]  SampleTime=-1  DataType=auto
      settings: SignalType=auto
  WindRates : Inport  Port=5  PortDimensions=[3 1]  SampleTime=-1  DataType=auto
      settings: SignalType=auto
  rho : Inport  Port=6  PortDimensions=1  SampleTime=-1  DataType=auto
      settings: SignalType=auto
  a : Inport  Port=7  PortDimensions=1  SampleTime=-1  DataType=auto
      settings: SignalType=auto
  AGL : Inport  Port=8  PortDimensions=1  SampleTime=-1  DataType=auto
      settings: SignalType=auto
  CGpos : Inport  Port=9  PortDimensions=[3 1]  SampleTime=-1  DataType=auto
      settings: SignalType=auto
  Gear : Inport  Port=10  PortDimensions=1  SampleTime=-1  DataType=auto
      settings: SignalType=auto
  Aerodynamic Force : aerosimlib/Aerodynamics/Aerodynamic Force  S=AC.Metrics.WingArea
  Aerodynamic Moment : aerosimlib/Aerodynamics/Aerodynamic Moment  c=AC.Metrics.WingChord  b=AC.Metrics.WingSpan  S=AC.Metrics.WingArea
  Drag : Subsystem  SimViewingDevice=off
      settings: Permissions=ReadWrite  RTWFcnNameOpts=Auto  RTWFileNameOpts=Auto
  Dynamic Pressure : aerosimlib/Aerodynamics/Dynamic Pressure
  Lift : Subsystem  SimViewingDevice=off
      settings: Permissions=ReadWrite  RTWFcnNameOpts=Auto  RTWFileNameOpts=Auto
  Mux : Mux  Inputs=6
  Pitch : Subsystem  SimViewingDevice=off
      settings: Permissions=ReadWrite  RTWFcnNameOpts=Auto  RTWFileNameOpts=Auto
  Roll : Subsystem  SimViewingDevice=off
      settings: Permissions=ReadWrite  RTWFcnNameOpts=Auto  RTWFileNameOpts=Auto
  Saturation : Saturate  UpperLimit=1  LowerLimit=0  LinearizeAsGain=on
  Side : Subsystem  SimViewingDevice=off
      settings: Permissions=ReadWrite  RTWFcnNameOpts=Auto  RTWFileNameOpts=Auto
  Sum : Sum  Inputs=|+-  SaturateOnIntegerOverflow=on
  Sum1 : Sum  Inputs=|+-  SaturateOnIntegerOverflow=on
  Sum2 : Sum  Inputs=|++  SaturateOnIntegerOverflow=on
  Wind-axes Velocities : aerosimlib/Aerodynamics/Wind-axes Velocities  Vabnd=[0 1000]  betabnd=[-1 1]  alphabnd=AC.Aerodynamics.AlphaLim
  Yaw : Subsystem  SimViewingDevice=off
      settings: Permissions=ReadWrite  RTWFcnNameOpts=Auto  RTWFileNameOpts=Auto
  h/b : Gain  Gain=1/AC.Metrics.WingSpan  Multiplication=Element-wise(K.*u)  SaturateOnIntegerOverflow=on
  r x F : aerosimlib/Math/Cross Product
  r_aero : Constant  Value=AC.Metrics.ACLoc
  Faero : Outport  Port=1
  Maero : Outport  Port=2
  AeroCoeff : Outport  Port=3
  VelW : Outport  Port=4
  pdyn : Outport  Port=5
  Mach : Outport  Port=6
  wires:
  Gear/1 -> Drag/3(Gear)
  r x F/1 -> Sum2/2
  Sum2/1 -> Maero/1
  Aerodynamic Moment/1 -> Sum2/1
  Sum1/1 -> r x F/1
  r_aero/1 -> Sum1/1
  CGpos/1 -> Sum1/2
  Rates/1 -> Sum/1
  Sum/1 -> Yaw/3(AngularRates), Pitch/4(AngularRates), Roll/3(AngularRates), Side/3(AngularRates), Lift/4(AngularRates)
  WindRates/1 -> Sum/2
  Saturation/1 -> Lift/5(GndEffect)
  AGL/1 -> h/b/1
  h/b/1 -> Saturation/1
  Wind-axes Velocities/3 -> Mach/1
  Aerodynamic Force/1 -> r x F/2, Faero/1
  Yaw/1(Cn) -> Mux/6, Aerodynamic Moment/3
  Pitch/1(Cm) -> Mux/5, Aerodynamic Moment/2
  Roll/1(Cl) -> Mux/4, Aerodynamic Moment/1
  Dynamic Pressure/1 -> pdyn/1, Aerodynamic Moment/4, Aerodynamic Force/4
  Side/1(CY) -> Mux/2, Aerodynamic Force/2
  Drag/1(CD) -> Mux/1, Aerodynamic Force/1
  Lift/1(CL) -> Mux/3, Aerodynamic Force/3
  Wind-axes Velocities/2 -> Lift/3(AlphaBetaDot), Pitch/3(AlphaBetaDot)
  Control/1 -> Pitch/1(Control), Yaw/1(Control), Roll/1(Control), Side/1(Control), Drag/1(Control), Lift/1(Control)
  Wind-axes Velocities/1 -> Lift/2(WindAxesVel), VelW/1, Aerodynamic Force/5, Yaw/2(WindAxesVel), Pitch/2(WindAxesVel), Roll/2(WindAxesVel), Side/2(WindAxesVel), Drag/2(WindAxesVel), Dynamic Pressure/1
  rho/1 -> Dynamic Pressure/2
  a/1 -> Wind-axes Velocities/3
  WindB/1 -> Wind-axes Velocities/2
  VelB/1 -> Wind-axes Velocities/1
  Mux/1 -> AeroCoeff/1

== system tp333079/FlightGear-Compatible/Complete Aircraft/CESSNA-310/Aircraft Inertia ==
  FuelFlow : Inport  Port=1  PortDimensions=-1  SampleTime=-1  DataType=auto
      settings: SignalType=auto
  RST : Inport  Port=2  PortDimensions=-1  SampleTime=-1  DataType=auto
      settings: SignalType=auto
  1/Ntank : Gain  Gain=1/length(AC.Propulsion.Tank)  Multiplication=Element-wise(K.*u)  SaturateOnIntegerOverflow=on
  Empty Aircraft : aerosimlib/FlightGear-Compatible/Inertia/Empty Aircraft  Metrics=AC.Metrics
  Left Inner Tank : aerosimlib/FlightGear-Compatible/Propulsion/Tank/Fuel Tank  MassIni=FuelIni(3)  Tank=AC.Propulsion.Tank{3}
  Left Outer Tank : aerosimlib/FlightGear-Compatible/Propulsion/Tank/Fuel Tank  MassIni=FuelIni(1)  Tank=AC.Propulsion.Tank{1}
  Product{,1..3,5} (5 alike) : Product  Inputs=2  Multiplication=Element-wise(.*)  SaturateOnIntegerOverflow=on
  Product4 : Product  Inputs=*/  Multiplication=Element-wise(.*)  SaturateOnIntegerOverflow=on
  Right Inner Tank : aerosimlib/FlightGear-Compatible/Propulsion/Tank/Fuel Tank  MassIni=FuelIni(4)  Tank=AC.Propulsion.Tank{4}
  Right Outer Tank : aerosimlib/FlightGear-Compatible/Propulsion/Tank/Fuel Tank  MassIni=FuelIni(2)  Tank=AC.Propulsion.Tank{2}
  Sum1 : Sum  Inputs=+++++  SaturateOnIntegerOverflow=on
  Sum2 : Sum  Inputs=+++++  SaturateOnIntegerOverflow=on
  Sum3 : Sum  Inputs=+++++  SaturateOnIntegerOverflow=on
  Mass : Outport  Port=1
  CG : Outport  Port=2
  Inertia : Outport  Port=3
  wires:
  Product5/1 -> Sum1/5
  Right Inner Tank/2 -> Product5/2
  Right Inner Tank/1 -> Sum2/5, Product5/1
  Right Inner Tank/3 -> Sum3/5
  Sum3/1 -> Inertia/1
  Left Inner Tank/3 -> Sum3/4
  Right Outer Tank/3 -> Sum3/3
  Left Outer Tank/3 -> Sum3/2
  Empty Aircraft/3 -> Sum3/1
  Product4/1 -> CG/1
  Sum1/1 -> Product4/1
  Product2/1 -> Sum1/4
  Product1/1 -> Sum1/3
  Product/1 -> Sum1/2
  Product3/1 -> Sum1/1
  Empty Aircraft/2 -> Product3/2
  Left Inner Tank/2 -> Product2/2
  Right Outer Tank/2 -> Product1/2
  Left Outer Tank/2 -> Product/2
  Left Inner Tank/1 -> Product2/1, Sum2/4
  Right Outer Tank/1 -> Product1/1, Sum2/3
  Left Outer Tank/1 -> Product/1, Sum2/2
  Empty Aircraft/1 -> Product3/1, Sum2/1
  Sum2/1 -> Product4/2, Mass/1
  RST/1 -> Left Outer Tank/2, Right Inner Tank/2, Left Inner Tank/2, Right Outer Tank/2
  FuelFlow/1 -> 1/Ntank/1
  1/Ntank/1 -> Right Inner Tank/1, Left Inner Tank/1, Left Outer Tank/1, Right Outer Tank/1

== system tp333079/FlightGear-Compatible/Complete Aircraft/CESSNA-310/Earth ==
  note: Inputs
  note: Outputs
  Position : Inport  Port=1  PortDimensions=[3 1]  SampleTime=-1  DataType=double
      settings: SignalType=auto
  EGM-96 : aerosimlib/Earth/EGM-96
  Ground Alt : Constant  Value=GndAlt
  Ground Detection : aerosimlib/Earth/Ground Detection
  Mux3 : Mux  Inputs=2
  WGS-84 : aerosimlib/Earth/WGS-84
  MSL : Outport  Port=1
  AGL : Outport  Port=2
  AConGnd : Outport  Port=3
  Rearth : Outport  Port=4
  Requiv : Outport  Port=5
  Gravity : Outport  Port=6
  wires:
  Position/1 -> EGM-96/1, WGS-84/1
  Ground Alt/1 -> Ground Detection/2
  EGM-96/1 -> Ground Detection/1, MSL/1
  WGS-84/1 -> Mux3/1
  WGS-84/2 -> Mux3/2
  Ground Detection/2 -> AGL/1
  Ground Detection/1 -> AConGnd/1
  Mux3/1 -> Rearth/1
  WGS-84/3 -> Requiv/1
  WGS-84/4 -> Gravity/1

== system tp333079/FlightGear-Compatible/Complete Aircraft/CESSNA-310/Equations of Motion ==
  note: Inputs
  note: Outputs
  Accel : Inport  Port=1  PortDimensions=[3 1]  SampleTime=-1  DataType=auto
      settings: SignalType=auto
  Moment : Inport  Port=2  PortDimensions=[3 1]  SampleTime=-1  DataType=auto
      settings: SignalType=auto
  Inertia : Inport  Port=3  PortDimensions=[4 1]  SampleTime=-1  DataType=auto
      settings: SignalType=auto
  Rearth : Inport  Port=4  PortDimensions=[2 1]  SampleTime=-1  DataType=auto
      settings: SignalType=auto
  Gravity : Inport  Port=5  PortDimensions=1  SampleTime=-1  DataType=auto
      settings: SignalType=auto
  AConGnd : Inport  Port=6  PortDimensions=1  SampleTime=-1  DataType=auto
      settings: SignalType=auto
  RST : Inport  Port=7  PortDimensions=1  SampleTime=-1  DataType=auto
      settings: SignalType=auto
  Angular Rate : aerosimlib/Equations of Motion/Geodetic-Frame EOM/Angular Rate  RatesIni=RatesIni
  Attitude (Quaternions) : aerosimlib/Equations of Motion/Body-Frame EOM/Kinematics (Quaternions)  QuaternionsIni=QuaternionsIni
  Body-Inertial DCM From Quaternions : aerosimlib/Transformations/Body-Inertial DCM From Quaternions
  Demux : Demux  Outputs=2  BusSelectionMode=off
  Euler Angles From Quaternions : aerosimlib/Transformations/Euler Angles From Quaternions
  Position : aerosimlib/Equations of Motion/Geodetic-Frame EOM/Position  PositionIni=PositionIni
  Product : Product  Inputs=2  Multiplication=Matrix(*)  SaturateOnIntegerOverflow=on
  Velocity : aerosimlib/Equations of Motion/Geodetic-Frame EOM/Velocity  VelocitiesIni=VelocitiesIni
  VelB : Outport  Port=1
  VelNED : Outport  Port=2
  Rates : Outport  Port=3
  Quaternions : Outport  Port=4
  Pos : Outport  Port=5
  DCM : Outport  Port=6
  Euler : Outport  Port=7
  Ang Acc : Outport  Port=8
  wires:
  Attitude (Quaternions)/1 -> Quaternions/1, Euler Angles From Quaternions/1, Body-Inertial DCM From Quaternions/1
  Position/1 -> Velocity/1, Angular Rate/3, Pos/1
  Position/2 -> Velocity/2, Angular Rate/4
  Velocity/1 -> Product/2, Position/1, VelNED/1
  Demux/1 -> Position/2
  Demux/2 -> Position/3
  Rearth/1 -> Demux/1
  Gravity/1 -> Velocity/5
  RST/1 -> Velocity/6, Position/5, Angular Rate/6, Attitude (Quaternions)/2
  Angular Rate/1 -> Rates/1, Attitude (Quaternions)/1
  Moment/1 -> Angular Rate/2
  Inertia/1 -> Angular Rate/1
  Body-Inertial DCM From Quaternions/1 -> Angular Rate/5, Velocity/4, Product/1, DCM/1
  AConGnd/1 -> Position/4
  Accel/1 -> Velocity/3
  Product/1 -> VelB/1
  Angular Rate/2 -> Ang Acc/1
  Euler Angles From Quaternions/1 -> Euler/1

== system tp333079/FlightGear-Compatible/Propulsion/Engine/Piston ==
  AirFlow Model : Subsystem  SimViewingDevice=off  mask(AirFlow){VolEff=VolEff, Disp=Displacement}
      mask prompts: VolEff "Volumetric efficiency:"; Disp "Engine displacement"
      mask help: Estimate the airflow to a JSBSim engine as a function of MAP, RPM, and atmospheric conditions.
      settings: Permissions=ReadWrite  RTWFcnNameOpts=Auto  RTWFileNameOpts=Auto
      mask Help:
      | Estimate the airflow to a JSBSim engine as a function of MAP, RPM, and atmospheric conditions.
      | <P><B>Inputs:</B>
      | <LI>MAP = the current manifold pressure</LI>
      | <LI>RPM = the current engine rotation speed</LI>
      | <LI>rho = the air density at current altitude</LI>
      | <LI>p = the current atmospheric pressure</LI>
      | </P>
      | <P><B>Outputs:</B>
      | <LI>Airflow = the mass airflow</LI>
      | </P>
      | <P><B>Parameters:</B>
      | <LI>Volumetric efficiency (approx. 0.8)</LI>
      | <LI>Engine displacement</LI>
      | </P>
  FG Piston Engine : Subsystem  SimViewingDevice=off  mask(FlightGear Piston Engine){Eng=Engine, pSL=pSL, TSL=TSL}
      mask prompts: Eng "Engine structure:"; pSL "Sea-level pressure:"; TSL "Sea-level temperature:"
      mask help: The FlightGear Piston Engine computes the engine power output, air and fuel flow as functions of engine control settings and atmospheric conditions.
      settings: Permissions=ReadWrite  RTWFcnNameOpts=Auto  RTWFileNameOpts=Auto
      mask Help:
      | The FlightGear Piston Engine computes the engine power output, air and fuel flow as functions of engine control settings and atmospheric conditions.
      | <P><B>Inputs:</B>
      | <LI>Thr = the current throttle fraction</LI>
      | <LI>Mix = the current air/fuel mixture setting</LI>
      | <LI>Omega = the current engine rotation speed</LI>
      | <LI>p = the atmospheric pressure</LI>
      | <LI>T = the outside-air temperature</LI>
      | <LI>rho = the air density at current altitude</LI>
      | </P>
      | <P><B>Outputs:</B>
      | <LI>MAP = the manifold pressure</LI>
      | <LI>AirFlow = the mass air flow</LI>
      | <LI>FuelFlow = the mass fuel flow</LI>
      | <LI>BSFC = the brake-specific fuel consumption</LI>
      | <LI>Power = the current power output</LI>
      | <LI>Torque = the torque delivered at engine shaft</LI>
      | </P>
      | <P><B>Parameters:</B>
      | <LI>Engine structure = a Matlab engine structure, which is part of the aircraft structure</LI>
      | <LI>The sea-level pressure and temperature for which the engine data is given.</LI>
      | </P>
  FuelFlow Model : Subsystem  SimViewingDevice=off  mask(FuelFlow){pSL=pSL}
      mask prompts: pSL "Sea-level ambient pressure:"
      mask help: Estimate the mass fuel flow to the engine as a function of mixture setting, airflow, and atmospheric conditions.
      settings: Permissions=ReadWrite  RTWFcnNameOpts=Auto  RTWFileNameOpts=Auto
      mask Help:
      | Estimate the mass fuel flow to the engine as a function of mixture setting, airflow, and atmospheric conditions.
      | <P><B>Inputs:</B>
      | <LI>Mix = the air/fuel mixture</LI>
      | <LI>p = the atmospheric pressure</LI>
      | <LI>AirFlow = the current mass airflow</LI>
      | </P>
      | <P><B>Outputs:</B>
      | <LI>EquivRatio = the equivalence ratio</LI>
      | <LI>FuelFlow = the mass fuel flow</LI>
      | </P>
      | <P><B>Parameters:</B>
      | <LI>Sea-level pressure</LI>
      | </P>
  Intake Model : Subsystem  SimViewingDevice=off  mask(Intake){MAPLim=MAPLim, pSL=pSL}
      mask prompts: MAPLim "MAP limits:"; pSL "Sea-level ambient pressure:"
      mask help: The block computes the manifold pressure as a function of throttle area fraction, atmosphere parameters and fuel flow.
      settings: Permissions=ReadWrite  RTWFcnNameOpts=Auto  RTWFileNameOpts=Auto
      mask Help:
      | The block computes the manifold pressure as a function of throttle area fraction, atmosphere parameters and fuel flow.
      | <P><B>Inputs:</B>
      | <LI>Thr = the current throttle fraction</LI>
      | <LI>p = the atmospheric pressure</LI>
      | </P>
      | <P><B>Outputs:</B>
      | <LI>MAP = the manifold pressure</LI>
      | </P>
      | <P><B>Parameters:</B>
      | <LI>MAP limits = the [min max] manifold pressure limits</LI>
      | <LI>Sea-level ambient pressure = the sea-level pressure for which the above MAP limits are given</LI>
      | </P>
  Power Model : Subsystem  SimViewingDevice=off  mask(Power){TSL=TSL, MaxPower=MaxPower, Mixture=MixVec, PowerMixCor=PwrMixVec}
      mask prompts: TSL "Sea-level ambient temperature:"; MaxPower "Maximum power:"; Mixture "Mixture vector:"; PowerMixCor "Power-mixture correlation:"
      mask help: Estimate the power output of a JSBSim piston engine as a function of MAP, RPM, and propellant mass flow.
      settings: Permissions=ReadWrite  RTWFcnNameOpts=Auto  RTWFileNameOpts=Auto
      mask Help:
      | Estimate the power output of a JSBSim piston engine as a function of MAP, RPM, and propellant mass flow.
      | <P><B>Inputs:</B>
      | <LI>MAP = the current manifold pressure</LI>
      | <LI>RPM = the current engine rotation speed</LI>
      | <LI>T = the outside air temperature</LI>
      | <LI>EquivRatio = the equivalence ratio</LI>
      | </P>
      | <P><B>Outputs:</B>
      | <LI>Power = the engine power output</LI>
      | </P>
      | <P><B>Parameters:</B>
      | <LI>Sea-level ambient temperature</LI>
      | <LI>Maximum power, at sea-level</LI>
      | <LI>Mixture vector = the mixture look-up table argument</LI>
      | <LI>Power-mixture correlation = look-up table for power-mixture correlation factor as a function of mixture</LI>
      | </P>

== system tp333079/FlightGear-Compatible/Propulsion/Tank/Fuel Tank ==
  MassFlow : Inport  Port=1  PortDimensions=-1  SampleTime=-1  DataType=auto
      settings: SignalType=auto
  RST : Inport  Port=2  PortDimensions=-1  SampleTime=-1  DataType=auto
      settings: SignalType=auto
  2/5 : Constant  Value=2/5
  ChSign : Gain  Gain=-1  Multiplication=Element-wise(K.*u)  SaturateOnIntegerOverflow=on
  Flow Integrator : Integrator  ExternalReset=rising  InitialConditionSource=internal  InitialCondition=MassIni  LimitOutput=on  UpperSaturationLimit=Tank.Capacity  LowerSaturationLimit=0  ShowSaturationPort=off  ShowStatePort=off  AbsoluteTolerance=auto
  J : Product  Inputs=3  Multiplication=Element-wise(.*)  SaturateOnIntegerOverflow=on
  J1 : Product  Inputs=2  Multiplication=Element-wise(.*)  SaturateOnIntegerOverflow=on
  J2 : Product  Inputs=2  Multiplication=Element-wise(.*)  SaturateOnIntegerOverflow=on
  J3 : Product  Inputs=2  Multiplication=Element-wise(.*)  SaturateOnIntegerOverflow=on
  Jxz : Product  Inputs=3  Multiplication=Element-wise(.*)  SaturateOnIntegerOverflow=on
  Math Function{,1..3} (4 alike) : Math  Operator=square  OutputSignalType=auto
  Mux : Mux  Inputs=3
  Mux1 : Mux  Inputs=4
  Radius : Constant  Value=Tank.Radius
  Sum{,1..5} (6 alike) : Sum  Inputs=++  SaturateOnIntegerOverflow=on
  x pos : Constant  Value=Tank.Loc(1)
  y pos : Constant  Value=Tank.Loc(2)
  z pos : Constant  Value=Tank.Loc(3)
  Mass : Outport  Port=1
  CG : Outport  Port=2
  Inertia : Outport  Port=3
  wires:
  Mux1/1 -> Inertia/1
  Jxz/1 -> Mux1/4
  Sum5/1 -> Mux1/3
  Sum4/1 -> Mux1/2
  Sum3/1 -> Mux1/1
  Mux/1 -> CG/1
  J3/1 -> Sum5/2
  J2/1 -> Sum4/2
  J1/1 -> Sum3/2
  J/1 -> Sum4/1, Sum5/1, Sum3/1
  Sum/1 -> J3/2
  Sum2/1 -> J2/2
  Sum1/1 -> J1/2
  Math Function3/1 -> Sum2/2, Sum1/2
  Math Function2/1 -> Sum1/1, Sum/2
  Math Function1/1 -> Sum2/1, Sum/1
  z pos/1 -> Math Function3/1, Mux/3, Jxz/3
  y pos/1 -> Mux/2, Math Function2/1
  x pos/1 -> Mux/1, Jxz/2, Math Function1/1
  Flow Integrator/1 -> Mass/1, J1/1, J2/1, J3/1, Jxz/1, J/1
  2/5/1 -> J/3
  Math Function/1 -> J/2
  Radius/1 -> Math Function/1
  RST/1 -> Flow Integrator/2
  MassFlow/1 -> ChSign/1
  ChSign/1 -> Flow Integrator/1
